simulink model "switch_5_24_comparator"  (R2016b)
settings: Solver=VariableStepAuto  StartTime=0.0  StopTime=0.001  RelTol=1e-3
libraries: fl_lib x10, nesl_utility x4, elec_lib x2
settings Model: Creator=piotr  LastModifiedBy=piotr

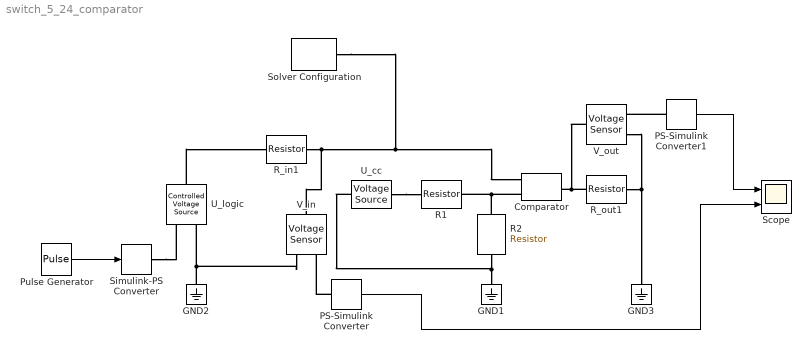
== system switch_5_24_comparator ==
  Comparator : elec_lib/Integrated Circuits/Comparator  V_OS=0.5 mV  V_OL=0 V  V_OH=24 V  C_IN=1.0 pF  R_OUT=50 Ohm  Delay=300 ns
  GND1 : fl_lib/Electrical/Electrical Elements/Electrical Reference
  GND2 : fl_lib/Electrical/Electrical Elements/Electrical Reference
  GND3 : fl_lib/Electrical/Electrical Elements/Electrical Reference
  PS-Simulink Converter : nesl_utility/PS-Simulink Converter  PhysicalDomain=network_engine_domain  SubClassName=ps_output  LeftPortType=input  RightPortType=output  PseudoPeriodic=off  Frequencies=[]  Unit=1  AffineConversion=off
  PS-Simulink Converter1 : nesl_utility/PS-Simulink Converter  PhysicalDomain=network_engine_domain  SubClassName=ps_output  LeftPortType=input  RightPortType=output  PseudoPeriodic=off  Frequencies=[]  Unit=1  AffineConversion=off
  Pulse Generator : DiscretePulseGenerator  PulseType=Time based  Amplitude=5.5  Period=0.0004  PulseWidth=50
  R1 : fl_lib/Electrical/Electrical Elements/Resistor  R=100 kOhm  i_specify=off  i_priority=None  i=0 A  v_specify=off  v_priority=None  v=0 V
  R2 : fl_lib/Electrical/Electrical Elements/Resistor  R=100 kOhm  i_specify=off  i_priority=None  i=0 A  v_specify=off  v_priority=None  v=0 V
  R_in1 : fl_lib/Electrical/Electrical Elements/Resistor  R=1 kOhm  i_specify=off  i_priority=None  i=0 A  v_specify=off  v_priority=None  v=0 V
  R_out1 : fl_lib/Electrical/Electrical Elements/Resistor  R=10 kOhm  i_specify=off  i_priority=None  i=0 A  v_specify=off  v_priority=None  v=0 V
  Scope : Scope  NumInputPorts=2
  Simulink-PS Converter : nesl_utility/Simulink-PS Converter  PhysicalDomain=network_engine_domain  SubClassName=ps_input  LeftPortType=input  RightPortType=output  PseudoPeriodic=off  Frequencies=[]  NoiseDistribution=none  NoiseParameters=[]  Unit=1  AffineConversion=off  InputFiltering=off  SimscapeFilterOrder=1  InputFilterTimeConstant=0.001  UdotUserProvided=1
  Solver Configuration : nesl_utility/Solver Configuration  PhysicalDomain=network_engine_domain  SubClassName=solver  LeftPortType=input  RightPortType=generic  Accelerate=off  Tones=[]  Harmonics=[]  SimulateNoise=off  Profile=off  UseLocalSampling=off  EnableSwitchedLinearOptims=on  FrequencyDomain=off  UseCCode=off  RelTol=0.001  AbsTol=1e-06  MinStep=1e-09  ToWorkspace=off  RevertToSquareIcSolve=off  NumHomotopyIterations=100  PhasorMode=off  PhasorModeNumHarmonics=1  OverrideAbsTol=off  DoDC=off  ResidualTolerance=1e-9  UseLocalSolver=off  LocalSolverChoice=NE_TRAPEZOIDAL_ADVANCER  LocalSolverSampleTime=0.0001  DoFixedCost=off  MaxNonlinIter=3  MaxModeIter=2  LinearAlgebra=Sparse  DelaysMemoryBudget=1024  AutomaticFiltering=on  FilteringTimeConstant=0.001
  U_cc : elec_lib/Sources/Voltage Source  dc_voltage=5.5 V  ac_voltage=0 V  ac_shift=0 deg  ac_frequency=60 Hz  noise_mode=0  PSD=0 V^2/Hz  sample_time=0.001 s  repeatability=1  auto_seed=1396490070  user_seed=0
  U_logic : fl_lib/Electrical/Electrical Sources/Controlled Voltage Source
  V_in : fl_lib/Electrical/Electrical Sensors/Voltage Sensor
  V_out : fl_lib/Electrical/Electrical Sensors/Voltage Sensor
  wires:
  Pulse Generator/1 -> Simulink-PS Converter/1
  PS-Simulink Converter1/1 -> Scope/1
  PS-Simulink Converter/1 -> Scope/2
  connections:
  U_logic/LConn1 -- R_in1/LConn1
  Simulink-PS Converter/RConn1 -- U_logic/RConn1
  Comparator/LConn2 -- R1/RConn1 -- R2/LConn1
  R2/RConn1 -- U_cc/RConn1 -- GND1/LConn1
  R_in1/RConn1 -- V_in/LConn1 -- Solver Configuration/RConn1 -- Comparator/LConn1
  U_cc/LConn1 -- R1/LConn1
  GND2/LConn1 -- V_in/RConn2 -- U_logic/RConn2
  R_out1/LConn1 -- V_out/LConn1 -- Comparator/RConn1
  R_out1/RConn1 -- V_out/RConn2 -- GND3/LConn1
  PS-Simulink Converter/LConn1 -- V_in/RConn1
  PS-Simulink Converter1/LConn1 -- V_out/RConn1
